simulink model "ModifiedHVDC"  (R2024b)
settings: Solver=ode3  StartTime=0.0  StopTime=2.5  FixedStep=7.4074074074074075E-6  RelTol=1e-3  AbsTol=1e-2
InitFcn:
  | Fnom = 50;        % Hz
  | 
  | Fc = 27*Fnom;   % (Hz)
  | Ts_Power = 1/(Fc*100);
  | Ts_Control = Ts_Power*10;
values from neighbouring files (symbols this model uses):
  C_per_km = 2.3100e-007    (= 2.31e-07)    [Parameters.m]
  L_per_km = 1.5900e-004    (= 0.000159)    [Parameters.m]
  L_total = 75    [Parameters.m]
  R_per_km = 1.3900e-002    (= 0.0139)    [Parameters.m]
  x_fault = 13    [Parameters.m]
undefined symbols (not defined in the file or in its folder): D1, Delta, DiscIntNeverNeededParam, magnitude
libraries: spsSecondOrderFilterLib x20, spsSeriesRLCBranchLib x14, spsMeanVariableFrequencyLib x12, spsabctoAlphaBetaZeroLib x8, spsThreePhaseVIMeasurementLib x6, spsAlphaBetaZerotodq0Lib x6, spsPiSectionLineLib x4, spsCurrentMeasurementLib x4, spsThreePhaseHarmonicFilterLib x4, spsVoltageMeasurementLib x4, spsFirstOrderFilterLib x4, spsGroundLib x3
(part 5 of 5)

== system ModifiedHVDC/VSC Controller Station 2/Discrete VSC Controller /Outer Active-Reactive Power and Voltage Loop/Reactive_Power_Control/AC Voltage Control Override  ==
  note: Reset states when enabling
  note: Override Regulator
  note: Active when input (In) is outside its range [min_in, max_in] otherwise the output goes back to zero
  In : Inport
  Enable (reset) : EnablePort  StatesWhenEnabling=reset  PropagateVarSize=During execution
  Add : Sum
  Constant1 : Constant  Value=max_in
  Constant2 : Constant  Value=min_in
  Constant3 : Constant  Value=Kp
  Discrete-Time Integrator1 : DiscreteIntegrator  IntegratorMethod=Integration: Trapezoidal  gainval=Ki  InitialCondition=IC_i  SampleTime=Ts  LimitOutput=on  UpperSaturationLimit=0  LowerSaturationLimit=min_out_lim  ICPrevOutput=DiscIntNeverNeededParam  ICPrevScaledInput=DiscIntNeverNeededParam
      settings: AttributesFormatString=Gain=%<gainval>\nMin=%<LowerSaturationLimit>\nMax=%<UpperSaturationLimit>
  Discrete-Time Integrator2 : DiscreteIntegrator  IntegratorMethod=Integration: Trapezoidal  gainval=Ki  InitialCondition=IC_i  SampleTime=Ts  LimitOutput=on  UpperSaturationLimit=max_out_lim  LowerSaturationLimit=0  ICPrevOutput=DiscIntNeverNeededParam  ICPrevScaledInput=DiscIntNeverNeededParam
      settings: AttributesFormatString=Gain=%<gainval>\nMin=%<LowerSaturationLimit>\nMax=%<UpperSaturationLimit>
  Product : Product  RndMeth=Zero
  Saturation : Saturate  UpperLimit=0  LowerLimit=min_out_lim
      settings: AttributesFormatString=Min=%<LowerLimit>\nMax=%<UpperLimit>
  Saturation1 : Saturate  UpperLimit=max_out_lim  LowerLimit=0
      settings: AttributesFormatString=Min=%<LowerLimit>\nMax=%<UpperLimit>
  Saturation2 : Saturate  UpperLimit=max_out_lim  LowerLimit=min_out_lim
      settings: AttributesFormatString=Min=%<LowerLimit>\nMax=%<UpperLimit>
  Subtract : Sum  Inputs=+-
  Subtract1 : Sum  Inputs=-+
  Sum2 : Sum  Inputs=+++  SaturateOnIntegerOverflow=on
  Out : Outport  VectorParamsAs1DForOutWhenUnconnected=off
  wires:
  Constant2/1 -> Subtract1/2
  Constant1/1 -> Subtract/1
  Discrete-Time Integrator2/1 -> Sum2/3  "positive"
  Discrete-Time Integrator1/1 -> Sum2/2  "negative"
  Product/1 -> Sum2/1
  Saturation1/1 -> Add/2
  Saturation/1 -> Add/1
  Add/1 -> Product/2
  Constant3/1 -> Product/1
  In/1 -> Subtract1/1, Subtract/2
  Subtract/1 -> Discrete-Time Integrator1/1, Saturation/1
  Subtract1/1 -> Saturation1/1, Discrete-Time Integrator2/1
  Sum2/1 -> Saturation2/1
  Saturation2/1 -> Out/1

== system ModifiedHVDC/VSC Controller Station 2/Discrete VSC Controller /Outer Active-Reactive Power and Voltage Loop/Reactive_Power_Control/Freeze_integrator ==
  note: Freeze Integrator
  note: Low AC voltage level
  U_meas : Inport
  Constant8 : Constant  Value=V_level_rpc
  Relational Operator : RelationalOperator  Operator=<=  InputSameDT=off
  Freeze : Outport  VectorParamsAs1DForOutWhenUnconnected=off
  wires:
  U_meas/1 -> Relational Operator/1
  Relational Operator/1 -> Freeze/1
  Constant8/1 -> Relational Operator/2

== system ModifiedHVDC/VSC Controller Station 2/Discrete VSC Controller /Outer Active-Reactive Power and Voltage Loop/Reactive_Power_Control/Int_regulator (type 1) ==
  note: Reset states when enabling
  note: Integral Regulator
      | (Type 1)
  Ord : Inport
  Meas : Inport  Port=2
  freeze : Inport  Port=3
  Enable (Reset) : EnablePort  StatesWhenEnabling=reset  PropagateVarSize=During execution
  Add : Sum
  Add1 : Sum
  Constant7 : Constant  Value=0.0
  Discrete-Time Integrator : DiscreteIntegrator  IntegratorMethod=Integration: Trapezoidal  gainval=Ki  InitialCondition=IC_i  SampleTime=Ts  LimitOutput=on  UpperSaturationLimit=max_i  LowerSaturationLimit=min_i  ICPrevOutput=DiscIntNeverNeededParam  ICPrevScaledInput=DiscIntNeverNeededParam
      settings: AttributesFormatString=Gain=%<gainval>\nMin=%<LowerSaturationLimit>\nMax=%<UpperSaturationLimit>
  Kf : Gain  Gain=Kf
      settings: AttributesFormatString=Gain=%<Gain>
  Saturation : Saturate  UpperLimit=max_out  LowerLimit=min_out
      settings: AttributesFormatString=Min=%<LowerLimit>\nMax=%<UpperLimit>
  Subtract : Sum  Inputs=+-
  Sum2 : Sum  Inputs=|+-  SaturateOnIntegerOverflow=on
  Switch : Switch  Criteria=u2 > Threshold  InputSameDT=off
  Unit Delay : UnitDelay  SampleTime=Ts_Control  HasFrameUpgradeWarning=on
      settings: AttributesFormatString=IC=%<InitialCondition>
  Out : Outport  VectorParamsAs1DForOutWhenUnconnected=off
  wires:
  Kf/1 -> Unit Delay/1
  Subtract/1 -> Switch/3
  Meas/1 -> Subtract/2
  Switch/1 -> Add/1
  Constant7/1 -> Switch/1
  freeze/1 -> Switch/2
  Discrete-Time Integrator/1 -> Add1/2
  Add1/1 -> Sum2/2, Saturation/1
  Sum2/1 -> Kf/1
  Ord/1 -> Subtract/1, Add1/1
  Add/1 -> Discrete-Time Integrator/1
  Unit Delay/1 -> Add/2
  Saturation/1 -> Sum2/1, Out/1

== system ModifiedHVDC/VSC Controller Station 1/Discrete VSC Controller /Outer Active-Reactive Power and Voltage Loop/Active_Power_Control/Ramping/Rate Limiter with external rates & reset (discrete) IC:0 ==
  note: Rate Limiter with external rates & reset (Discrete)
  note: IC=ic
  note: Max= 4
      | Min =1
  note: Silvano Casoria
      | IREQ
  In : Inport
  up_rate : Inport  Port=2
  down_rate : Inport  Port=3
  R : Inport  Port=4
  Abs : Abs
  Constant3 : Constant
  Data Type Conversion1 : DataTypeConversion
  Data Type Conversion2 : DataTypeConversion
  Data Type Conversion3 : DataTypeConversion
  Gain1 : Gain  Gain=2  SaturateOnIntegerOverflow=on  OutDataTypeStr=Inherit: Same as input  ParamDataTypeStr=Inherit: Same as input
  Gain2 : Gain  Gain=3  SaturateOnIntegerOverflow=on  OutDataTypeStr=Inherit: Same as input  ParamDataTypeStr=Inherit: Same as input
  Gain3 : Gain  Gain=st  SaturateOnIntegerOverflow=on  OutDataTypeStr=Inherit: Same as input  ParamDataTypeStr=Inherit: Same as input
  Gain4 : Gain  Gain=-st  SaturateOnIntegerOverflow=on  OutDataTypeStr=Inherit: Same as input  ParamDataTypeStr=Inherit: Same as input
  Multiport Switch : MultiPortSwitch  Inputs=4
  Relational Operator : RelationalOperator  Operator=>
  Relational Operator2 : RelationalOperator  Operator=<
  Saturation : Saturate  UpperLimit=4  LowerLimit=1
  Sum : Sum  Inputs=+-  InputSameDT=on  SaturateOnIntegerOverflow=on  OutDataTypeStr=Inherit: Same as first input
  Sum1 : Sum  Inputs=++++  InputSameDT=on  SaturateOnIntegerOverflow=on  OutDataTypeStr=Inherit: Same as first input
  Sum2 : Sum  InputSameDT=on  SaturateOnIntegerOverflow=on  OutDataTypeStr=Inherit: Same as first input
  Sum3 : Sum  InputSameDT=on  SaturateOnIntegerOverflow=on  OutDataTypeStr=Inherit: Same as first input
  Unit Delay : UnitDelay  InitialCondition=ic  SampleTime=st  HasFrameUpgradeWarning=on
  " " : Outport  InitialOutput=0  VectorParamsAs1DForOutWhenUnconnected=off
  wires:
  Gain2/1 -> Sum1/3
  Constant3/1 -> Sum1/4
  Relational Operator/1 -> Data Type Conversion2/1
  Gain1/1 -> Sum1/2
  Saturation/1 -> Multiport Switch/1
  Sum1/1 -> Saturation/1
  R/1 -> Data Type Conversion3/1
  Sum3/1 -> Multiport Switch/4
  Sum2/1 -> Multiport Switch/3
  In/1 -> Multiport Switch/5, Multiport Switch/2, Sum/1
  Relational Operator2/1 -> Data Type Conversion1/1
  Sum/1 -> Relational Operator2/1, Relational Operator/1  "Rate"
  Multiport Switch/1 -> " "/1, Unit Delay/1
  Gain4/1 -> Sum3/2, Relational Operator2/2
  Gain3/1 -> Sum2/2, Relational Operator/2
  Unit Delay/1 -> Sum3/1, Sum2/1, Sum/2
  up_rate/1 -> Gain3/1
  down_rate/1 -> Abs/1
  Abs/1 -> Gain4/1
  Data Type Conversion1/1 -> Gain1/1
  Data Type Conversion2/1 -> Sum1/1
  Data Type Conversion3/1 -> Gain2/1

== system ModifiedHVDC/VSC Controller Station 2/Discrete VSC Controller /Outer Active-Reactive Power and Voltage Loop/Active_Power_Control/Ramping/Rate Limiter with external rates & reset (discrete) IC:0 ==
  note: Rate Limiter with external rates & reset (Discrete)
  note: IC=ic
  note: Max= 4
      | Min =1
  note: Silvano Casoria
      | IREQ
  In : Inport
  up_rate : Inport  Port=2
  down_rate : Inport  Port=3
  R : Inport  Port=4
  Abs : Abs
  Constant3 : Constant
  Data Type Conversion1 : DataTypeConversion
  Data Type Conversion2 : DataTypeConversion
  Data Type Conversion3 : DataTypeConversion
  Gain1 : Gain  Gain=2  SaturateOnIntegerOverflow=on  OutDataTypeStr=Inherit: Same as input  ParamDataTypeStr=Inherit: Same as input
  Gain2 : Gain  Gain=3  SaturateOnIntegerOverflow=on  OutDataTypeStr=Inherit: Same as input  ParamDataTypeStr=Inherit: Same as input
  Gain3 : Gain  Gain=st  SaturateOnIntegerOverflow=on  OutDataTypeStr=Inherit: Same as input  ParamDataTypeStr=Inherit: Same as input
  Gain4 : Gain  Gain=-st  SaturateOnIntegerOverflow=on  OutDataTypeStr=Inherit: Same as input  ParamDataTypeStr=Inherit: Same as input
  Multiport Switch : MultiPortSwitch  Inputs=4
  Relational Operator : RelationalOperator  Operator=>
  Relational Operator2 : RelationalOperator  Operator=<
  Saturation : Saturate  UpperLimit=4  LowerLimit=1
  Sum : Sum  Inputs=+-  InputSameDT=on  SaturateOnIntegerOverflow=on  OutDataTypeStr=Inherit: Same as first input
  Sum1 : Sum  Inputs=++++  InputSameDT=on  SaturateOnIntegerOverflow=on  OutDataTypeStr=Inherit: Same as first input
  Sum2 : Sum  InputSameDT=on  SaturateOnIntegerOverflow=on  OutDataTypeStr=Inherit: Same as first input
  Sum3 : Sum  InputSameDT=on  SaturateOnIntegerOverflow=on  OutDataTypeStr=Inherit: Same as first input
  Unit Delay : UnitDelay  InitialCondition=ic  SampleTime=st  HasFrameUpgradeWarning=on
  " " : Outport  InitialOutput=0  VectorParamsAs1DForOutWhenUnconnected=off
  wires:
  Gain2/1 -> Sum1/3
  Constant3/1 -> Sum1/4
  Relational Operator/1 -> Data Type Conversion2/1
  Gain1/1 -> Sum1/2
  Saturation/1 -> Multiport Switch/1
  Sum1/1 -> Saturation/1
  R/1 -> Data Type Conversion3/1
  Sum3/1 -> Multiport Switch/4
  Sum2/1 -> Multiport Switch/3
  In/1 -> Multiport Switch/5, Multiport Switch/2, Sum/1
  Relational Operator2/1 -> Data Type Conversion1/1
  Sum/1 -> Relational Operator2/1, Relational Operator/1  "Rate"
  Multiport Switch/1 -> " "/1, Unit Delay/1
  Gain4/1 -> Sum3/2, Relational Operator2/2
  Gain3/1 -> Sum2/2, Relational Operator/2
  Unit Delay/1 -> Sum3/1, Sum2/1, Sum/2
  up_rate/1 -> Gain3/1
  down_rate/1 -> Abs/1
  Abs/1 -> Gain4/1
  Data Type Conversion1/1 -> Gain1/1
  Data Type Conversion2/1 -> Sum1/1
  Data Type Conversion3/1 -> Gain2/1
